simulink model "lv_new_test"  (Simulink 7.1)
settings: Solver=ode45  StartTime=0.0  StopTime=1000  RelTol=1e-3
values from neighbouring files (symbols this model uses):
  C1 = 0.44    [lv_demofile.m]    (also in lv_demofile1.m; lv_demofile2.m; lv_demofile4.m; lv_demofile5.m)
  C2 = 0.0167    [lv_demofile.m]    (also in lv_demofile1.m; lv_demofile2.m; lv_demofile4.m; lv_demofile5.m)
  C3 = 0.3    [lv_demofile.m]    (also in lv_demofile1.m; lv_demofile2.m; lv_demofile4.m; lv_demofile5.m)
  C4 = 0.00184    [lv_demofile.m]    (also in lv_demofile1.m; lv_demofile2.m; lv_demofile4.m; lv_demofile5.m)
  Jem = 90    [lv_cankaofile.m]    (also in lv_demofile.m = 97.5; lv_demofile1.m = 97.5; lv_demofile2.m = 97.5; lv_demofile3.m = 97.5)
  Jwt = 9e7    (= 90000000)    [lv_cankaofile.m]    (also in lv_demofile.m = 3275300; lv_demofile1.m = 3275300; lv_demofile2.m = 3275300; lv_demofile3.m = 3275300)
  K = 83    [lv_cankaofile.m]    (also in lv_demofile.m; lv_demofile1.m = 75.76; lv_demofile2.m; lv_demofile3.m = 75.76)
  R = 40    [lv_cankaofile.m]    (also in lv_demofile.m = 38.5; lv_demofile1.m = 38.75; lv_demofile2.m = 38.5; lv_demofile3.m = 38.5)
  ro_air = 1.225    [lv_cankaofile.m]    (also in lv_demofile.m = 1.2236; lv_demofile1.m; lv_demofile2.m = 1.2236; lv_demofile3.m)
libraries: simulink x1, wt_blockset_v3 x1
settings Model: Creator=lv  LastModifiedBy=lv

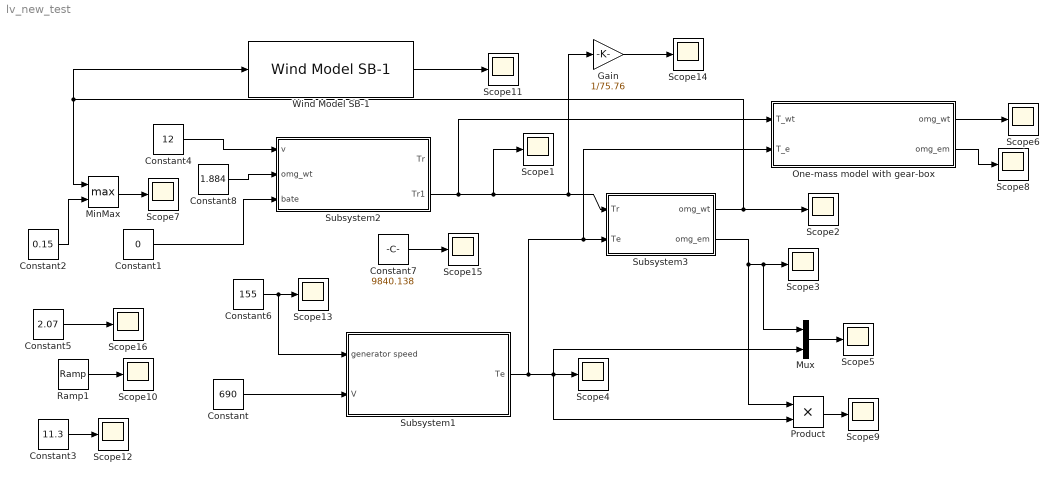
== system lv_new_test ==
  Constant : Constant  Value=690  OutDataType=sfix(16)  OutScaling=2^0
  Constant1 : Constant  Value=0  OutDataType=sfix(16)  OutScaling=2^0
  Constant2 : Constant  Value=0.15  OutDataType=sfix(16)  OutScaling=2^0
  Constant3 : Constant  Value=11.3  OutDataType=sfix(16)  OutScaling=2^0
  Constant4 : Constant  Value=12  OutDataType=sfix(16)  OutScaling=2^0
  Constant5 : Constant  Value=2.07  OutDataType=sfix(16)  OutScaling=2^0
  Constant6 : Constant  Value=155  OutDataType=sfix(16)  OutScaling=2^0
  Constant7 : Constant  Value=9840.138  OutDataType=sfix(16)  OutScaling=2^0
  Constant8 : Constant  Value=1.884  OutDataType=sfix(16)  OutScaling=2^0
  Gain : Gain  Gain=1/75.76  ParameterDataType=sfix(16)  ParameterScaling=2^0  OutDataType=sfix(16)  OutScaling=2^0
  MinMax : MinMax  Function=max  Inputs=2  OutDataType=sfix(16)  OutScaling=2^0
  Mux : Mux  Inputs=2
  One-mass model with gear-box : Subsystem  AncestorBlock=wt_blockset_v3/Mechanical Components/One-mass model with gear-box  mask(Simple Gearbox){Jem=Jem, Jwt=Jwt, K=K, init_speed=1.514}
      mask prompts: Jem "Electric machinery - Moment of inertia [kg m2]"; Jwt "Wind turbine rotor - Moment of inertia [kg*m2]"; K "Gearbox ratio"; init_speed "Initial condition [omg_wt (rad/sec)]"
      mask init:
      | J=Jem*K^2+Jwt;
      mask Display: disp('E M\nGear box')
  Product : Product  OutDataType=sfix(16)  OutScaling=2^0  RndMeth=Zero
  Ramp1 : simulink/Sources/Ramp  SystemSampleTime=-1  slope=0.5  start=0  X0=0
  Scope{1..16} (16 alike) : Scope
      Scope1 settings: TimeRange=1000  YMin=482185  YMax=482185
      Scope10 settings: TimeRange=12  YMin=-3e+010  YMax=5e+010  SaveName=ScopeData23
      Scope11 settings: TimeRange=1000  YMin=9  YMax=17.5  SaveName=ScopeData26
      Scope12 settings: TimeRange=12  YMin=-3e+010  YMax=5e+010  SaveName=ScopeData27
      Scope13 settings: TimeRange=12  YMin=-3e+010  YMax=5e+010  SaveName=ScopeData28
      Scope14 settings: TimeRange=1000  YMin=9309.33  YMax=9309.33  SaveName=ScopeData29
      Scope15 settings: TimeRange=12  YMin=-3e+010  YMax=5e+010  SaveName=ScopeData30
      Scope16 settings: TimeRange=12  YMin=-3e+010  YMax=5e+010  SaveName=ScopeData31
      Scope2 settings: TimeRange=12  YMin=-180.5  YMax=-173  SaveName=ScopeData2
      Scope3 settings: TimeRange=12  YMin=187.5  YMax=187.5  SaveName=ScopeData3
      Scope4 settings: TimeRange=12  YMin=-96.5  YMax=-91.5  SaveName=ScopeData5
      Scope5 settings: TimeRange=12  YMin=0  YMax=7500  SaveName=ScopeData17
      Scope6 settings: TimeRange=12  YMin=-10000  YMax=1000  SaveName=ScopeData19
      Scope7 settings: TimeRange=12  YMin=-3e+010  YMax=5e+010  SaveName=ScopeData18
      Scope8 settings: TimeRange=12  YMin=-10000  YMax=1000  SaveName=ScopeData24
      Scope9 settings: TimeRange=12  YMin=-4.8e+008  YMax=-4.6e+008  SaveName=ScopeData22
  Subsystem1 : Subsystem
  Subsystem2 : Subsystem
  Subsystem3 : Subsystem
  Wind Model SB-1 : wt_blockset_v3/Mechanical Components/Wind Model SB-1  SystemSampleTime=-1  D_rotor=77  v_mean=12  roughness=600  turb_int=12  T_sample=0.01
  wires:
  Constant1/1 -> Subsystem2/3(bate)
  Subsystem3/1(omg_wt) -> Scope2/1, Wind Model SB-1/1, MinMax/1
  Subsystem3/2(omg_em) -> Scope3/1, Mux/1, Product/1
  Constant/1 -> Subsystem1/2(V)
  Subsystem1/1(Te) -> Scope4/1, Product/2, Mux/2, Subsystem3/2(Te), One-mass model with gear-box/2(T_e)
  Product/1 -> Scope9/1
  Ramp1/1 -> Scope10/1
  Constant2/1 -> MinMax/2
  Mux/1 -> Scope5/1
  MinMax/1 -> Scope7/1
  One-mass model with gear-box/1(omg_wt) -> Scope6/1
  One-mass model with gear-box/2(omg_em) -> Scope8/1
  Subsystem2/2(Tr1) -> Scope1/1, Subsystem3/1(Tr), Gain/1, One-mass model with gear-box/1(T_wt)
  Wind Model SB-1/1 -> Scope11/1
  Constant3/1 -> Scope12/1
  Constant4/1 -> Subsystem2/1(v)
  Constant6/1 -> Scope13/1, Subsystem1/1(generator speed)
  Gain/1 -> Scope14/1
  Constant7/1 -> Scope15/1
  Constant5/1 -> Scope16/1
  Constant8/1 -> Subsystem2/2(omg_wt)

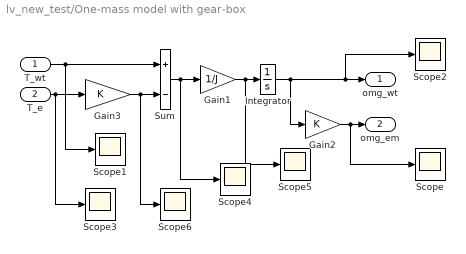
== system lv_new_test/One-mass model with gear-box ==
  T_wt : Inport  OutDataType=sfix(16)  OutScaling=2^0
  T_e : Inport  Port=2  OutDataType=sfix(16)  OutScaling=2^0
  Gain1 : Gain  Gain=1/J  ParameterDataType=sfix(16)  ParameterScaling=2^0  OutDataType=sfix(16)  OutScaling=2^0  SaturateOnIntegerOverflow=on  OutDataTypeStr=Inherit: Same as input  ParamDataTypeStr=Inherit: Same as input
  Gain2 : Gain  Gain=K  ParameterDataType=sfix(16)  ParameterScaling=2^0  OutDataType=sfix(16)  OutScaling=2^0  SaturateOnIntegerOverflow=on  OutDataTypeStr=Inherit: Same as input  ParamDataTypeStr=Inherit: Same as input
  Gain3 : Gain  Gain=K  ParameterDataType=sfix(16)  ParameterScaling=2^0  OutDataType=sfix(16)  OutScaling=2^0  SaturateOnIntegerOverflow=on  OutDataTypeStr=Inherit: Same as input  ParamDataTypeStr=Inherit: Same as input
  Integrator : Integrator  InitialCondition=init_speed  UpperSaturationLimit=0.95*2*pi*60  LowerSaturationLimit=0
  Scope{,1..6} (7 alike) : Scope
      Scope settings: TimeRange=10  SaveName=ScopeData20
      Scope1 settings: TimeRange=10  SaveName=ScopeData24
      Scope2 settings: YMin=-2.25e+010  YMax=1.5e+010  SaveName=ScopeData21
      Scope3 settings: TimeRange=10  SaveName=ScopeData25
      Scope4 settings: TimeRange=10  YMin=-1.5e+006  YMax=1.5e+006  SaveName=ScopeData2
      Scope5 settings: TimeRange=10  SaveName=ScopeData22
      Scope6 settings: TimeRange=10  SaveName=ScopeData2
  Sum : Sum  Inputs=+-  OutDataType=sfix(16)  OutScaling=2^0  SaturateOnIntegerOverflow=on  InputSameDT=on  OutDataTypeStr=Inherit: Same as first input
  omg_wt : Outport  OutDataType=sfix(16)  OutScaling=2^0  InitialOutput=0
  omg_em : Outport  Port=2  OutDataType=sfix(16)  OutScaling=2^0  InitialOutput=0
  wires:
  Gain3/1 -> Sum/2, Scope6/1
  Gain2/1 -> omg_em/1, Scope/1
  Integrator/1 -> Gain2/1, omg_wt/1, Scope2/1
  T_wt/1 -> Sum/1, Scope1/1
  T_e/1 -> Gain3/1, Scope3/1
  Sum/1 -> Gain1/1, Scope4/1
  Gain1/1 -> Integrator/1, Scope5/1

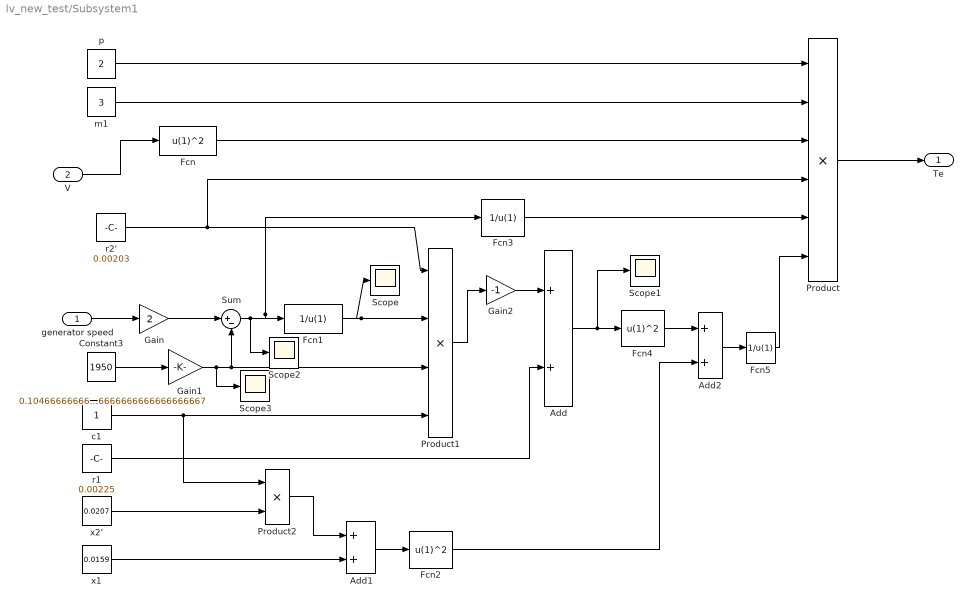
== system lv_new_test/Subsystem1 ==
  generator speed : Inport  OutDataType=sfix(16)  OutScaling=2^0
  V : Inport  Port=2  OutDataType=sfix(16)  OutScaling=2^0
  Add : Sum  OutDataType=sfix(16)  OutScaling=2^-10
  Add1 : Sum  OutDataType=sfix(16)  OutScaling=2^-10
  Add2 : Sum  OutDataType=sfix(16)  OutScaling=2^-10
  Constant3 : Constant  Value=1950  OutDataType=sfix(16)  OutScaling=2^0
  Fcn : Fcn  Expr=u(1)^2
  Fcn1 : Fcn  Expr=1/u(1)
  Fcn2 : Fcn  Expr=u(1)^2
  Fcn3 : Fcn  Expr=1/u(1)
  Fcn4 : Fcn  Expr=u(1)^2
  Fcn5 : Fcn  Expr=1/u(1)
  Gain : Gain  Gain=2  ParameterDataType=sfix(16)  ParameterScaling=2^0  OutDataType=sfix(16)  OutScaling=2^0
  Gain1 : Gain  Gain=0.10466666666666666666666666666667  ParameterDataType=sfix(16)  ParameterScaling=2^0  OutDataType=sfix(16)  OutScaling=2^0
  Gain2 : Gain  Gain=-1  ParameterDataType=sfix(16)  ParameterScaling=2^0  OutDataType=sfix(16)  OutScaling=2^0
  Product : Product  Inputs=6  OutDataType=sfix(16)  OutScaling=2^0  RndMeth=Zero
  Product1 : Product  Inputs=4  OutDataType=sfix(16)  OutScaling=2^0  RndMeth=Zero
  Product2 : Product  OutDataType=sfix(16)  OutScaling=2^0  RndMeth=Zero
  Scope{,1..3} (4 alike) : Scope
      Scope settings: YMin=0  YMax=100000  SaveName=ScopeData10
      Scope1 settings: YMin=0  YMax=100000  SaveName=ScopeData11
      Scope2 settings: YMin=0  YMax=100000  SaveName=ScopeData15
      Scope3 settings: YMin=0  YMax=100000  SaveName=ScopeData9
  Sum : Sum  Inputs=|+-  OutDataType=sfix(16)  OutScaling=2^0
  c1 : Constant  OutDataType=sfix(16)  OutScaling=2^0
  m1 : Constant  Value=3  OutDataType=sfix(16)  OutScaling=2^0
  p : Constant  Value=2  OutDataType=sfix(16)  OutScaling=2^0
  r1 : Constant  Value=0.00225  OutDataType=sfix(16)  OutScaling=2^0
  r2' : Constant  Value=0.00203  OutDataType=sfix(16)  OutScaling=2^0
  x1 : Constant  Value=0.0159  OutDataType=sfix(16)  OutScaling=2^0
  x2' : Constant  Value=0.0207  OutDataType=sfix(16)  OutScaling=2^0
  Te : Outport  OutDataType=sfix(16)  OutScaling=2^0
  wires:
  Fcn1/1 -> Scope/1, Product1/2
  Product/1 -> Te/1
  Fcn5/1 -> Product/6
  Add2/1 -> Fcn5/1
  Fcn2/1 -> Add2/2
  Fcn4/1 -> Add2/1
  Add/1 -> Scope1/1, Fcn4/1
  Fcn3/1 -> Product/5
  Gain2/1 -> Add/1
  r1/1 -> Add/2
  Fcn/1 -> Product/3
  m1/1 -> Product/2
  p/1 -> Product/1
  Product1/1 -> Gain2/1
  Add1/1 -> Fcn2/1
  x1/1 -> Add1/2
  Product2/1 -> Add1/1
  x2'/1 -> Product2/2
  c1/1 -> Product2/1, Product1/4
  r2'/1 -> Product/4, Product1/1
  Sum/1 -> Scope2/1, Fcn1/1, Fcn3/1
  Gain1/1 -> Product1/3, Sum/2, Scope3/1
  Constant3/1 -> Gain1/1
  Gain/1 -> Sum/1
  generator speed/1 -> Gain/1
  V/1 -> Fcn/1

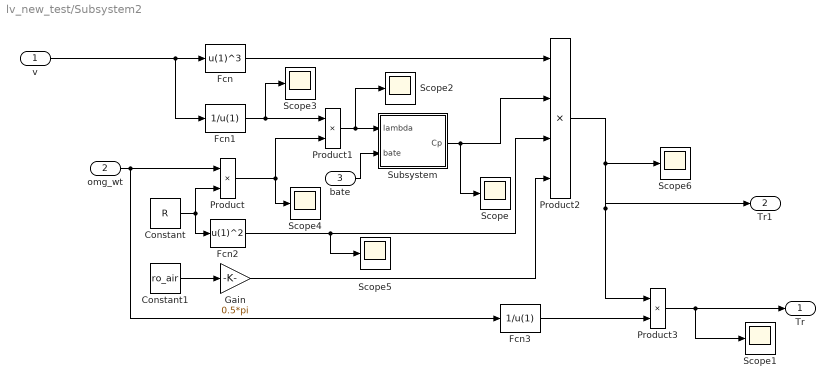
== system lv_new_test/Subsystem2 ==
  v : Inport  OutDataType=sfix(16)  OutScaling=2^0
  omg_wt : Inport  Port=2  OutDataType=sfix(16)  OutScaling=2^0
  bate : Inport  Port=3  OutDataType=sfix(16)  OutScaling=2^0
  Constant : Constant  Value=R  OutDataType=sfix(16)  OutScaling=2^0
  Constant1 : Constant  Value=ro_air  OutDataType=sfix(16)  OutScaling=2^0
  Fcn : Fcn  Expr=u(1)^3
  Fcn1 : Fcn  Expr=1/u(1)
  Fcn2 : Fcn  Expr=u(1)^2
  Fcn3 : Fcn  Expr=1/u(1)
  Gain : Gain  Gain=0.5*pi  ParameterDataType=sfix(16)  ParameterScaling=2^0  OutDataType=sfix(16)  OutScaling=2^0
  Product : Product  OutDataType=sfix(16)  OutScaling=2^0  RndMeth=Zero
  Product1 : Product  OutDataType=sfix(16)  OutScaling=2^0  RndMeth=Zero
  Product2 : Product  Inputs=4  OutDataType=sfix(16)  OutScaling=2^0  RndMeth=Zero
  Product3 : Product  OutDataType=sfix(16)  OutScaling=2^0  RndMeth=Zero
  Scope{,1..6} (7 alike) : Scope
      Scope settings: TimeRange=50  YMin=0.1772981595092024  YMax=0.2028981595092024  SaveName=ScopeData4
      Scope1 settings: TimeRange=20  YMin=-1500000  YMax=1500000
      Scope2 settings: SaveName=ScopeData6
      Scope3 settings: SaveName=ScopeData7
      Scope4 settings: SaveName=ScopeData8
      Scope5 settings: YMin=1426.48  YMax=1576.64  SaveName=ScopeData20
      Scope6 settings: TimeRange=20  YMin=-500000  YMax=5e+006  SaveName=ScopeData21
  Subsystem : Subsystem
  Tr : Outport  OutDataType=sfix(16)  OutScaling=2^0
  Tr1 : Outport  Port=2  OutDataType=sfix(16)  OutScaling=2^0
  wires:
  v/1 -> Fcn/1, Fcn1/1
  omg_wt/1 -> Product/1, Fcn3/1
  Constant/1 -> Product/2, Fcn2/1
  Fcn1/1 -> Product1/1, Scope3/1
  Product/1 -> Product1/2, Scope4/1
  Product1/1 -> Subsystem/1(lambda), Scope2/1
  bate/1 -> Subsystem/2(bate)
  Fcn/1 -> Product2/1
  Subsystem/1(Cp) -> Product2/2, Scope/1
  Fcn2/1 -> Product2/3, Scope5/1
  Gain/1 -> Product2/4
  Constant1/1 -> Gain/1
  Product2/1 -> Scope6/1, Product3/1, Tr1/1
  Fcn3/1 -> Product3/2
  Product3/1 -> Scope1/1, Tr/1

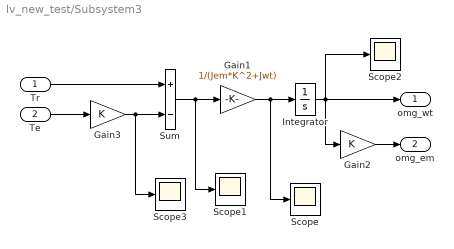
== system lv_new_test/Subsystem3 ==
  Tr : Inport  OutDataType=sfix(16)  OutScaling=2^0
  Te : Inport  Port=2  OutDataType=sfix(16)  OutScaling=2^0
  Gain1 : Gain  Gain=1/(Jem*K^2+Jwt)  ParameterDataType=sfix(16)  ParameterScaling=2^0  OutDataType=sfix(16)  OutScaling=2^0  SaturateOnIntegerOverflow=on  OutDataTypeStr=Inherit: Same as input  ParamDataTypeStr=Inherit: Same as input
  Gain2 : Gain  Gain=K  ParameterDataType=sfix(16)  ParameterScaling=2^0  OutDataType=sfix(16)  OutScaling=2^0  SaturateOnIntegerOverflow=on  OutDataTypeStr=Inherit: Same as input  ParamDataTypeStr=Inherit: Same as input
  Gain3 : Gain  Gain=K  ParameterDataType=sfix(16)  ParameterScaling=2^0  OutDataType=sfix(16)  OutScaling=2^0  SaturateOnIntegerOverflow=on  OutDataTypeStr=Inherit: Same as input  ParamDataTypeStr=Inherit: Same as input
  Integrator : Integrator  InitialCondition=1.884  UpperSaturationLimit=2.5  LowerSaturationLimit=0
  Scope{,1..3} (4 alike) : Scope
      Scope settings: YMin=-0.0125373  YMax=-0.0125373  SaveName=ScopeData12
      Scope1 settings: YMin=-47939.2  YMax=-47939.2  SaveName=ScopeData13
      Scope2 settings: YMin=-1  YMax=1  SaveName=ScopeData14
      Scope3 settings: YMin=721903  YMax=721903  SaveName=ScopeData16
  Sum : Sum  Inputs=+-  OutDataType=sfix(16)  OutScaling=2^0  SaturateOnIntegerOverflow=on  InputSameDT=on  OutDataTypeStr=Inherit: Same as first input
  omg_wt : Outport  OutDataType=sfix(16)  OutScaling=2^0  InitialOutput=0
  omg_em : Outport  Port=2  OutDataType=sfix(16)  OutScaling=2^0  InitialOutput=0
  wires:
  Gain1/1 -> Integrator/1, Scope/1
  Sum/1 -> Gain1/1, Scope1/1
  Te/1 -> Gain3/1
  Tr/1 -> Sum/1
  Gain2/1 -> omg_em/1
  Gain3/1 -> Sum/2, Scope3/1
  Integrator/1 -> omg_wt/1, Gain2/1, Scope2/1

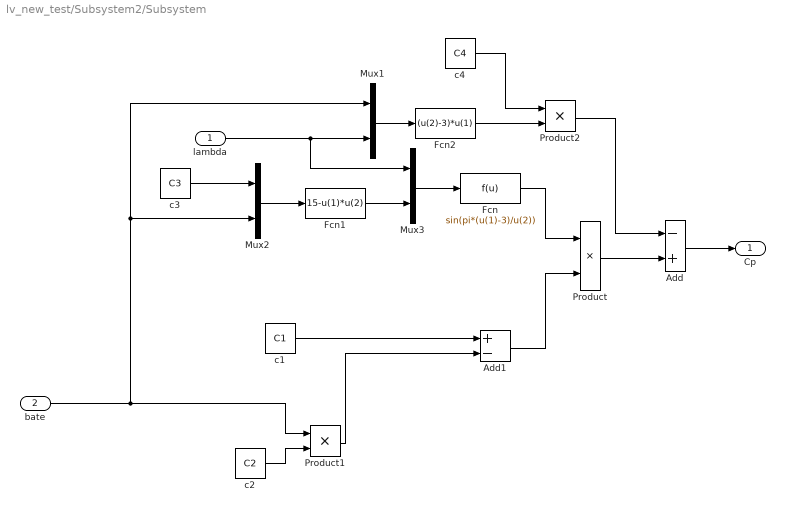
== system lv_new_test/Subsystem2/Subsystem ==
  lambda : Inport  OutDataType=sfix(16)  OutScaling=2^0
  bate : Inport  Port=2  OutDataType=sfix(16)  OutScaling=2^0
  Add : Sum  Inputs=-+  OutDataType=sfix(16)  OutScaling=2^-10
  Add1 : Sum  Inputs=+-  OutDataType=sfix(16)  OutScaling=2^-10
  Fcn : Fcn  Expr=sin(pi*(u(1)-3)/u(2))
  Fcn1 : Fcn  Expr=15-u(1)*u(2)
  Fcn2 : Fcn  Expr=(u(2)-3)*u(1)
  Mux1 : Mux  Inputs=2
  Mux2 : Mux  Inputs=2
  Mux3 : Mux  Inputs=2
  Product : Product  OutDataType=sfix(16)  OutScaling=2^0  RndMeth=Zero
  Product1 : Product  OutDataType=sfix(16)  OutScaling=2^0  RndMeth=Zero
  Product2 : Product  OutDataType=sfix(16)  OutScaling=2^0  RndMeth=Zero
  c1 : Constant  Value=C1  OutDataType=sfix(16)  OutScaling=2^0
  c2 : Constant  Value=C2  OutDataType=sfix(16)  OutScaling=2^0
  c3 : Constant  Value=C3  OutDataType=sfix(16)  OutScaling=2^0
  c4 : Constant  Value=C4  OutDataType=sfix(16)  OutScaling=2^0
  Cp : Outport  OutDataType=sfix(16)  OutScaling=2^0
  wires:
  Add/1 -> Cp/1
  Product2/1 -> Add/1
  Fcn2/1 -> Product2/2
  c4/1 -> Product2/1
  Mux1/1 -> Fcn2/1
  lambda/1 -> Mux1/2, Mux3/1
  Fcn1/1 -> Mux3/2
  Product/1 -> Add/2
  Add1/1 -> Product/2
  Fcn/1 -> Product/1
  Mux3/1 -> Fcn/1
  c3/1 -> Mux2/1
  Mux2/1 -> Fcn1/1
  Product1/1 -> Add1/2
  c2/1 -> Product1/2
  bate/1 -> Mux1/1, Mux2/2, Product1/1
  c1/1 -> Add1/1
